simulink model "automata_learning"  (Simulink 9.1)
settings: Solver=VariableStepAuto  StartTime=0.0  StopTime=10.0  RelTol=1e-3
settings Model: Creator=xiaodong  LastModifiedBy=xiaodong
settings DataIOCC: SaveFormat=Dataset
settings OptimizationCC: LifeSpan=auto
settings DebuggingCC: UnderspecifiedInitializationDetection=Simplified  MergeDetectMultiDrivingBlocksExec=error  SFUnexpectedBacktrackingDiag=error  SFNoUnconditionalDefaultTransitionDiag=error  SFExecutionAtInitializationDiag=warning
settings HardwareCC: ProdBitPerPointer=64  ProdBitPerSizeT=64  ProdBitPerPtrDiffT=64  ProdLargestAtomicFloat=Float  ProdIntDivRoundTo=Zero  ProdEndianess=LittleEndian  ProdWordSize=64  ProdHWDeviceType=Intel->x86-64 (Windows64)
settings ModelReferenceCC: PropagateSignalLabelsOutOfModel=on
settings CodeAppCC: StateflowObjectComments=off
settings GRTTargetCC: TargetLangStandard=C99 (ISO)  CombineOutputUpdateFcns=on  GRTInterface=off
settings ConfigComp: CovMetricSettings=dwe  CovHtmlReporting=off  CovSaveCumulativeToWorkspaceVar=off  CovSaveSingleToWorkspaceVar=off  CovExternalEMLEnable=on

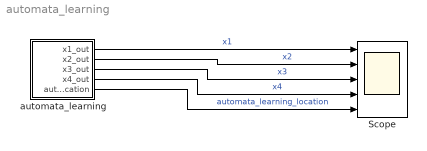
== system automata_learning ==
  Scope : Scope  NumInputPorts=5
  automata_learning : Stateflow chart  TreatAsAtomicUnit=on
  wires:
  automata_learning/1(x1_out) -> Scope/1  "x1"
  automata_learning/2(x2_out) -> Scope/2  "x2"
  automata_learning/3(x3_out) -> Scope/3  "x3"
  automata_learning/4(x4_out) -> Scope/4  "x4"
  automata_learning/5(automata_learning_location) -> Scope/5  "automata_learning_location"

== stateflow chart automata_learning ==
  settings: updateMethod=CONTINUOUS
  state loc1
    du:
    x1_dot = 0.0000000014426455294075608 * x2 - 0.0000000006780914427086392 * x1 + 1.0000002048473107 * x3 - 0.00000012488698096545583 * x4 - 0.000000154857611769834;
    x2_dot = 0.000000005180447670190551 * x2 - 0.000000002435121859100623 * x1 + 0.0000003634908525215752 * x3 + 0.9999997631857696 * x4 - 0.00000021754967455918026;
    x3_dot = 0.005986177435161721 * x1 - 0.012734982565689279 * x2 - 1.208034314069664 * x3 + 0.09938623106449995 * x4 + 1.2070961723329674;
    x4_dot = 0.01746719104079375 * x1 - 0.037159669219249736 * x2 + 0.07655670578628815 * x3 - 1.2017910254617163 * x4 - 0.07929416646948084;
    x1_out=x1;
    x2_out=x2;
    x3_out=x3;
    x4_out=x4;
    automata_learning_location =1;
  state loc2
    du:
    x1_dot = 0.000000000000010316211919236548 * x2 - 0.00000000000008618674401024362 * x1 + 1.0000000742220436 * x3 - 0.0000000182751270854601 * x4 - 0.00000001827514557538974;
    x2_dot = 0.0000000000000008246170640003595 * x2 - 0.00000000000006457400296023534 * x1 - 0.000000018275142992657534 * x3 + 1.0000000742220436 * x4 + 0.00000007422372897921727;
    x3_dot = 0.00000000000000000009442668241800939 * x1 - 0.000000000000016248046627159078 * x2 - 1.200000090895628 * x3 + 0.10000002935248631 * x4 + 0.10000002935248631;
    x4_dot = 0.10000002935248631 * x3 - 0.0000000000000027641430754330486 * x2 - 0.0000000000000000000944266813068988 * x1 - 1.200000090895628 * x4 - 1.200000090895628;
    x1_out=x1;
    x2_out=x2;
    x3_out=x3;
    x4_out=x4;
    automata_learning_location =2;
  state loc3
    du:
    x1_dot = 0.00000000000004083620250991668 * x2 - 0.00000000000002220446049250313 * x1 + 1.0000000742220436 * x3 - 0.000000018275139300135985 * x4 - 0.00000006540656826846576;
    x2_dot = 1.0000000742220436 * x4 - 0.000000018275084667080093 * x3 - 0.00000000000004856848414619176 * x2 + 0.00000006540656353115279;
    x3_dot = 0.000000000000013115232680016072 * x2 - 1.200000090895628 * x3 + 0.10000002935248631 * x4 + 0.9192389005711448;
    x4_dot = 0.10000002935248631 * x3 - 0.0000000000000093662809997335 * x2 - 1.200000090895628 * x4 - 0.9192389005711448;
    x1_out=x1;
    x2_out=x2;
    x3_out=x3;
    x4_out=x4;
    automata_learning_location =3;
  state loc4
    du:
    x1_dot = 0.00000000000004083620250991668 * x2 - 0.00000000000002220446049250313 * x1 + 1.0000000742220436 * x3 - 0.000000018275139300135985 * x4 - 0.00000006540656826846576;
    x2_dot = 1.0000000742220436 * x4 - 0.000000018275084667080093 * x3 - 0.00000000000004856848414619176 * x2 + 0.00000006540656353115279;
    x3_dot = 0.000000000000013115232680016072 * x2 - 1.200000090895628 * x3 + 0.10000002935248631 * x4 + 0.9192389005711448;
    x4_dot = 0.10000002935248631 * x3 - 0.0000000000000093662809997335 * x2 - 1.200000090895628 * x4 - 0.9192389005711448;
    x1_out=x1;
    x2_out=x2;
    x3_out=x3;
    x4_out=x4;
    automata_learning_location =4;
  state loc5
    du:
    x1_dot = 0.00000000000004083620250991668 * x2 - 0.00000000000002220446049250313 * x1 + 1.0000000742220436 * x3 - 0.000000018275139300135985 * x4 - 0.00000006540656826846576;
    x2_dot = 1.0000000742220436 * x4 - 0.000000018275084667080093 * x3 - 0.00000000000004856848414619176 * x2 + 0.00000006540656353115279;
    x3_dot = 0.000000000000013115232680016072 * x2 - 1.200000090895628 * x3 + 0.10000002935248631 * x4 + 0.9192389005711448;
    x4_dot = 0.10000002935248631 * x3 - 0.0000000000000093662809997335 * x2 - 1.200000090895628 * x4 - 0.9192389005711448;
    x1_out=x1;
    x2_out=x2;
    x3_out=x3;
    x4_out=x4;
    automata_learning_location =5;
  loc2 -> loc5 [order 3] : [0.005433 * x1 - 0.971 * x2 - 0.01764 * x3 + 0.05212 * x4 + 1.0 > 0.0]
  loc3 -> loc2 [order 2] : [0.001934 * x2 - 0.4784 * x1 - 0.04486 * x3 + 0.01677 * x4 + 1.0 < 0.0]
  loc1 -> loc2 [order 1] : [0.004247202660636162 * x1 - 0.9986482097065164 * x2 - 0.01149780050363347 * x3 + 0.021322810592096175 * x4 + 1.0 < 0.0 && 0.0029928459686701103 * x4 - 0.004893838521041971 * x2 - 0.0009215688441379655 * x3 - 0.49042439656386705 * x1 + 1.0 < 0.0]
  loc2 -> loc3 [order 1] : [0.003186 * x2 - 1.007 * x1 + 0.02068 * x3 - 0.002852 * x4 + 1.0 < 0.0]
  (default) -> loc1 : {x1 = 0.0;
      | x2 = 0.0;
      | x3 = 0.0;
      | x4 = 0.0;}
  loc2 -> loc1 [order 2] : [0.06652 * x1 - 0.6434 * x2 - 0.7096 * x3 + 0.5528 * x4 + 1.0 > 0.0]
  loc3 -> loc1 [order 1] : [0.2753 * x3 - 0.8002 * x2 - 0.09344 * x1 + 0.7353 * x4 + 1.0 < 0.0]
  loc1 -> loc4 [order 2] : [0.006683 * x3 - 0.0009015 * x2 - 0.5018 * x1 - 0.002991 * x4 + 1.0 < 0.0]
  data: x1_out output double; x1 local double; x2_out output double; x2 local double; x3_out output double; x3 local double; x4_out output double; x4 local double; automata_learning_location output double
  data x1 settings: updateMethod=SF_CONTINUOUS_TIME_DATA
  data x2 settings: updateMethod=SF_CONTINUOUS_TIME_DATA
  data x3 settings: updateMethod=SF_CONTINUOUS_TIME_DATA
  data x4 settings: updateMethod=SF_CONTINUOUS_TIME_DATA
